simulink model "NonLinearPlantModel"  (R2024a)
settings: Solver=VariableStepAuto  StartTime=0.0  StopTime=10  RelTol=1e-3
model workspace (MAT data in the model file):
  g = Simulink.Parameter
  g.Value = 9.80665
  g.Complexity = 'real'
  g.Dimensions = [1 1]
  g.DataType = 'auto'
  l = Simulink.Parameter
  l.Value = 3.60710863407
  l.Complexity = 'real'
  l.Dimensions = [1 1]
  l.DataType = 'auto'
settings Model: Creator=Riley  LastModifiedBy=Riley
settings DataIOCC: ExternalInput=crane_data.getElement('hoist_speed'),crane_data.getElement('crane_position')  LoadExternalInput=on

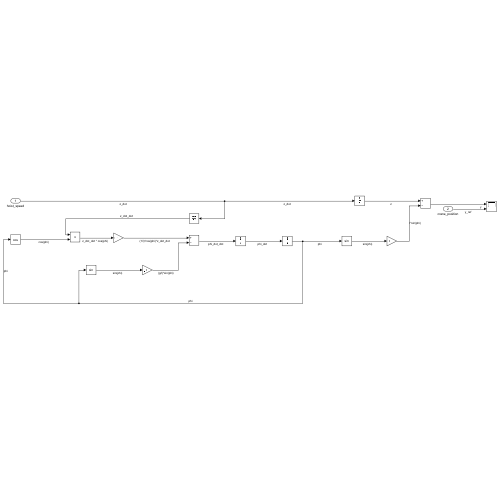
[thumbnail: Simulink's stored preview of the top-level diagram]
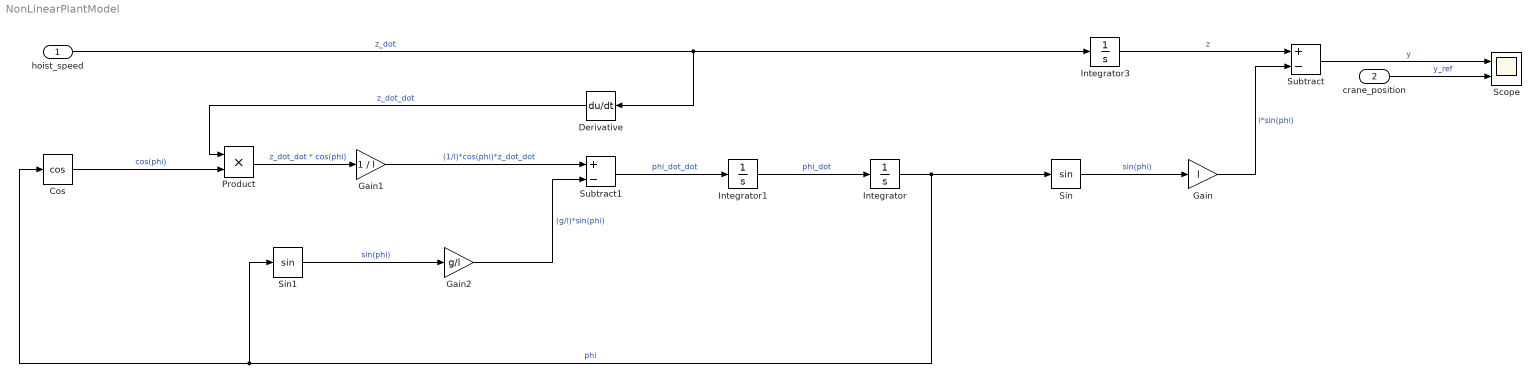
== system NonLinearPlantModel ==
  hoist_speed : Inport
  crane_position : Inport  Port=2
  Cos : Trigonometry  Operator=cos
  Derivative : Derivative
  Gain : Gain  Gain=l
  Gain1 : Gain  Gain=1 / l
  Gain2 : Gain  Gain=g/l
  Integrator : Integrator
  Integrator1 : Integrator
  Integrator3 : Integrator
  Product : Product
  Scope : Scope  NumInputPorts=2
  Sin : Trigonometry
  Sin1 : Trigonometry
  Subtract : Sum  Inputs=+-
  Subtract1 : Sum  Inputs=+-
  wires:
  Subtract/1 -> Scope/1  "y"
  Integrator3/1 -> Subtract/1  "z"
  Gain/1 -> Subtract/2  "l*sin(phi)"
  Sin/1 -> Gain/1  "sin(phi)"
  Integrator/1 -> Sin1/1, Cos/1, Sin/1  "phi"
  Integrator1/1 -> Integrator/1  "phi_dot"
  Subtract1/1 -> Integrator1/1  "phi_dot_dot"
  Derivative/1 -> Product/1  "z_dot_dot"
  Gain1/1 -> Subtract1/1  "(1/l)*cos(phi)*z_dot_dot"
  Cos/1 -> Product/2  "cos(phi)"
  Product/1 -> Gain1/1  "z_dot_dot * cos(phi)"
  Sin1/1 -> Gain2/1  "sin(phi)"
  Gain2/1 -> Subtract1/2  "(g/l)*sin(phi)"
  hoist_speed/1 -> Derivative/1, Integrator3/1  "z_dot"
  crane_position/1 -> Scope/2  "y_ref"
